simulink model "passThrough"  (R2023a)
settings: Solver=FixedStepDiscrete  StartTime=0.0  StopTime=100  RelTol=1e-3
InitFcn:
  | xlEvaluateHDLBlocks('passThrough')
undefined symbols (not defined in the file): S, vsva2197, xcvc1902
libraries: aieUtilities x2, hdlUtilities x2, aieBasic x1, simulink x1, hdlBasic x1, dspsrcs4 x1, vmcUtilities x1
settings Model: Creator=shirazi  LastModifiedBy=robg
settings SolverCC: AlgebraicLoopSolver=TrustRegion
settings DebuggingCC: UnconnectedInputMsg=warning  UnconnectedOutputMsg=warning  UnconnectedLineMsg=warning
settings ModelReferenceCC: EnableRefExpFcnMdlSchedulingChecks=on
settings SFSimCC: CustomCodeUndefinedFunction=UseInterfaceOnly
settings RTWCC: DLArmComputeVersion=19.05

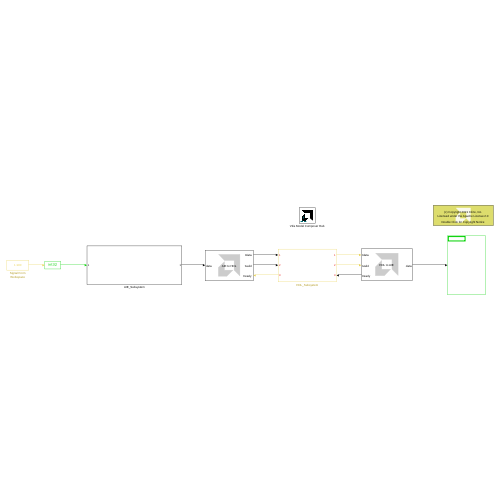
[thumbnail: Simulink's stored preview of the top-level diagram]
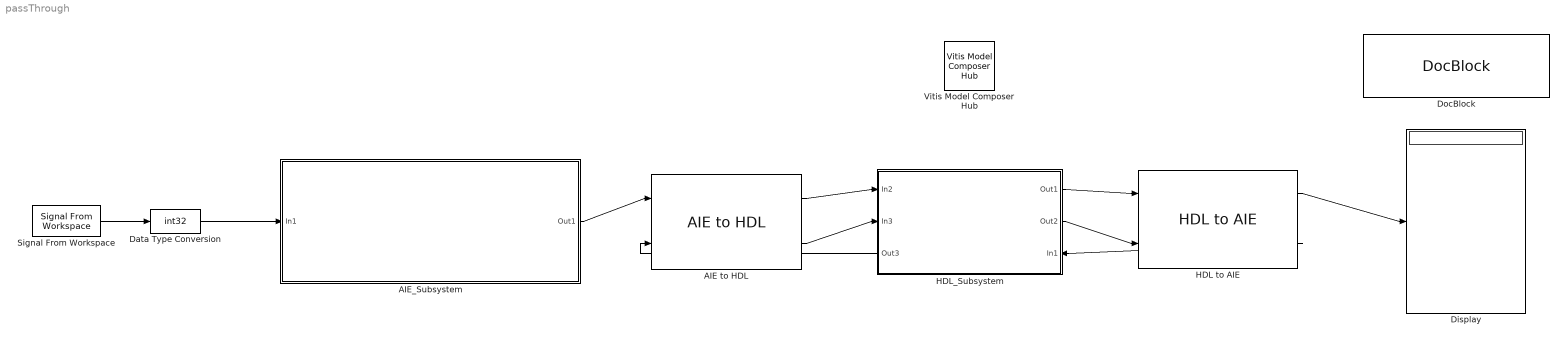
== system passThrough ==
  AIE to HDL : aieUtilities/AIE to HDL  OutDataType=int32  OutSampleTime=Inherit: Same as tready
  AIE_Subsystem : Subsystem
  Data Type Conversion : DataTypeConversion  OutDataTypeStr=int32  SaturateOnIntegerOverflow=off  RndMeth=Floor
  Display : Display
  DocBlock : simulink/Model-Wide Utilities/DocBlock  DocumentType=Text  mask(DocBlock){}
      content=|
      | ///////////////////////////////////////////////////////////////////////////
      | // Copyright 2021 Xilinx
      | //
      | // Licensed under the Apache License, Version 2.0 (the "License");
      | // you may not use this file except in compliance with the License.
      | // You may obtain a copy of the License at
      | //
      | // http://www.apache.org/licenses/LICENSE-2.0
      | //
      | // Unless required by applicable law or agreed to in writing, software
      | // distributed under the License is distributed on an "AS IS" BASIS,
      | // WITHOUT WARRANTIES OR CONDITIONS OF ANY KIND, either express or implied.
      | // See the License for the specific language governing permissions and
      | // limitations under the License.
      | ///////////////////////////////////////////////////////////////////////////
      mask Display:
      | xmcDrawBlockIcon();
      | disp(['{\fontsize{10pt}(c) Copyright 2021' ' Xilinx, Inc.}\newline \newline '],'texmode','on');
      | disp('{\fontsize{10pt}Licensed under the Apache License 2.0}','texmode','on');
      | disp('\newline \newline \newline{\fontsize{10pt}Double Click for Copyright Notice}','texmode','on');
  HDL to AIE : aieUtilities/HDL to AIE  InDataType=uint32  OutDataType=int32  OutSampleTime=1  SamplesPerFrame=8  RateReduceFactor=1  ManuallySpecifyOutSampleTime=on
  HDL_Subsystem : Subsystem
      settings: PortSchema="{\"entries\":[{\"content\":{\"sides\":[{\"content\":{\"connectorIds\":[\"In1\",\"In2\",\"Out3\"]},\"type\":\"ConnectorPlacement.EquallySpacedRectSide\",\"uuid\":\"989cb16a-31ef-4a7b-a4d3-adb9fa6297fb\"},{\"content\":{\"connectorIds\":[\"Out1\",\"Out2\",\"In3\"],\"side\":\"RIGHT\"},\"type\":\"ConnectorPlacement.EquallySpacedRectSide\",\"uuid\":\"9f541dfa-b9f2-4468-aad7-758d6944575e\"},{\"content\":{\"connectorIds\":[],\"side\":\"TOP\"},\"type\":\"ConnectorPlacement.EquallySpacedRectSide\",\"uuid\":\"c3c29352-583e-46d2-970b-15c15d07c124\"}]},\"type\":\"ConnectorPlacement.EquallySpacedConnector\",\"uuid\":\"c80158a0-6c2e-4236-83b1-850c61320738\"}],\"packageUris\":[\"http://schema.mathworks.com/mf0/Connector/19700101\"],\"version\":\"1.0\"}"
  Signal From Workspace : dspsrcs4/Signal From Workspace  X=1:100  Ts=1  nsamps=8  OutputAfterFinalValue=Cyclic repetition  ignoreOrWarnInputAndFrameLengths=off  OutputFrames=off
  Vitis Model Composer Hub : vmcUtilities/Vitis Model Composer Hub  Tag=genX  CodeGeneration=off  SubsystemName=AIE_Subsystem  StartColumn=1  NumberOfColumns=1  TargetDirectory=./code  exportDesign=off  analyzeDesign=off  validateDesignOnHw=off  ExportType=AI Engines  IpVendor=xilinx.com  IpLibrary=hls  IpVersion=1.0  IpHWLanguage=Verilog  AieCompilerOptions={}  AieSimulatorOptions={}  CreateTestbench=off  TestbenchStackSize=10  RunRtlSim=off  RunCSim=off  RunAieSim=off  AieSimTimeout=50000  RunAieSimProfiling=off  LaunchVitisAnalyzer=off  PlotOutput=off  RunX86Sim=off  X86SimTimeout=10  GenHwImage=off  GenLibadfXo=off  GenHwValidationCode=off  PlatformType=Not Specified  HwSystemType=Baremetal  HwValidationTarget=hw  ProjDevice=xcvc1902-vsva2197-1LP-e-S  ProjDevicePart=xcvc1902-vsva2197-1LP-e-S  AIEType=AIE  SamplePeriod=-1  ClockFrequency=200  DataPathParallelism=1  xilinxfamily=versalaicore  part=xcvc1902  speed=-1LP-e-S  package=vsva2197  directory=./netlist  testbench=off  incr_netlist=off  synthesis_tool=Vivado  clock_wrapper=Clock Enables  dbl_ovrd=According to Block Masks  dcm_input_clock_period=10  sysclk_period=10  simulink_period=1  eval_field=0  LogFileName=''  NThreads=4
  wires:
  Signal From Workspace/1 -> Data Type Conversion/1
  HDL to AIE/1 -> Display/1
  HDL_Subsystem/1(Out1) -> HDL to AIE/1
  AIE to HDL/1 -> HDL_Subsystem/1(In2)
  HDL_Subsystem/2(Out2) -> HDL to AIE/2
  AIE to HDL/2 -> HDL_Subsystem/2(In3)
  HDL to AIE/2 -> HDL_Subsystem/3(In1)
  HDL_Subsystem/3(Out3) -> AIE to HDL/2
  Data Type Conversion/1 -> AIE_Subsystem/1(In1)
  AIE_Subsystem/1(Out1) -> AIE to HDL/1

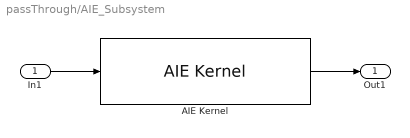
== system passThrough/AIE_Subsystem ==
  In1 : Inport
  AIE Kernel : aieBasic/AIE Kernel  KernelAllAttrs=s[12;12;9;9;19;14;21;23;24;21;12;24;26;26;26;27;28;9;21;23;23;23;24;25;14;19;19;29]@FunctionNameDeclFileNamePortNamesPortTypesPortSerializedTypesPortDirectionsPortWindowSizeEnablesPortWindowMarginEnablesPortSynchronicityEnablesPortSignalSizeEnablesFunctionDeclFunctionTemplateSpecKindFunctionTemplateParamNamesFunctionTemplateParamKindsFunctionTemplateParamTypesFunctionTemplateParamValuesFunctionTemplateParamEnablesClassDeclClassTemplateSpecKindClassTemplateParamNamesClassTemplateParamKindsClassTemplateParamTypesClassTemplateParamValuesClassTemplateParamEnablesClassCtorDeclsClassCtorParamNamesClassCtorParamTypesClassCtorParamSerializedTypes[1 1]@C[28 1]@t8@mysquaret16@../../mysquare.hC[2 1]@t3@in1t4@out1C[2 1]@t20@input_window_int32 *t21@output_window_int32 *C[2 1]@t30@{P{Tinput_window{1{t{Bi32}}}}}t31@{P{Toutput_window{1{t{Bi32}}}}}C[2 1]@t5@inputt6@outputC[2 1]@l1@l1@C[2 1]@l1@l0@C[2 1]@l1@l1@C[2 1]@l0@l0@t67@void mysquare(input_window_int32 * in1, output_window_int32 * out1)t4@nonee[0 1]@e[0 1]@e[0 1]@e[0 1]@e[0 1]@nne[0 1]@e[0 1]@e[0 1]@e[0 1]@e[0 1]@e[0 1]@e[0 1]@e[0 1]@e[0 1]@  PortNames={'in1'; 'out1'}  PortSerializedTypes={'{P{Tinput_window{1{t{Bi32}}}}}'; '{P{Toutput_window{1{t{Bi32}}}}}'}  PortWindowSizes={8.000000000000000000e+00, 8.000000000000000000e+00}  PortWindowMargins={0.000000000000000000e+00, 0.000000000000000000e+00}  PortSynchronicities={'sync', 'sync'}  PortSignalSizes={0.000000000000000000e+00; 0.000000000000000000e+00}  FunctionTemplateSpecKind=none  FunctionTemplateParamNames={}  FunctionTemplateParamKinds={}  FunctionTemplateParamTypes={}  FunctionTemplateParamValues={}  FunctionIndex=1  FunctionTabVisible=on  FunctionTemplateParamsVisible=off  FunctionDeclTypeOptions=C[1 1]@t70@void mysquare(input_window_int32 * _arg0, output_window_int32 * _arg1)  FunctionDecl=void mysquare(input_window_int32 * _arg0, output_window_int32 * _arg1)  FunctionTemplateParams={}  FunctionTemplateParamsEnables={}  PortAttrs={ 'Input', '_arg0', 'input_window_int32 *', '8', '0', 'sync', ''; 'Output', '_arg1', 'output_window_int32 *', '8', '', 'sync', '' }  PortAttrsEnables={'off', 'off', 'off', 'on', 'on', 'on', 'off';'off', 'off', 'off', 'on', 'off', 'on', 'off'}  SampleTime=-1  KernelHeaderFile=mysquare.h  KernelFunction=mysquare  KernelSourceFile=mysquare.cc  KernelSearchPaths={}  PreProcOptions={}  blockJsonConstraints=[]
  Out1 : Outport
  wires:
  In1/1 -> AIE Kernel/1
  AIE Kernel/1 -> Out1/1

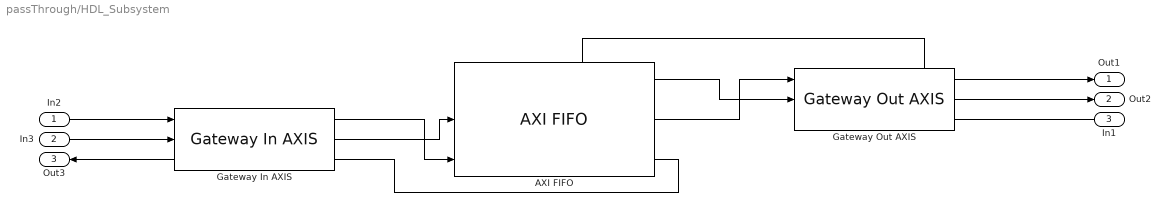
== system passThrough/HDL_Subsystem ==
  In2 : Inport
  In3 : Inport  Port=2
  In1 : Inport  Port=3
  AXI FIFO : hdlBasic/AXI FIFO  input_depth_axis=1K  actual_fifo_depth_label=1026  enable_tdata=on  enable_tdest=off  enable_tstrb=off  enable_tready=on  enable_tid=off  enable_tuser=off  enable_tkeep=off  enable_tlast=off  has_aresetn=off  enable_data_counts_axis=off  fifo_implementation_type_axis=Common Clock Block RAM  trim_axipin_name=off  programmable_full_type_axis=Full  full_threshold_assert_value_axis=0  programmable_empty_type_axis=Empty  empty_threshold_assert_value_axis=1022  underflow_flag_axi=0  underflow_sense_axi=Active High  overflow_flag_axi=0  overflow_sense_axi=Active High  simulation_type=fast_sim  XmcBlockStatus=1  maskContainerNames=tabcontainer1  block_type=axi_fifo  block_config=sysgen:AXI_FIFO_config
  Gateway In AXIS : hdlUtilities/Gateway In AXIS  gui_display_data_type=Fixed-point  arith_type=Signed (2's comp)  n_bits=32  bin_pt=0  preci_type=Custom  exp_width=16  frac_width=24  quantization=Truncate  overflow=Flag as error  OutSampleTime=1  block_type=gatewayinaxi  XmcBlockStatus=1
  Gateway Out AXIS : hdlUtilities/Gateway Out AXIS  mask_sample_period=1  block_type=gatewayoutaxi
  Out1 : Outport
  Out2 : Outport  Port=2
  Out3 : Outport  Port=3
  wires:
  AXI FIFO/2 -> Gateway Out AXIS/1
  AXI FIFO/1 -> Gateway Out AXIS/2
  In1/1 -> Gateway Out AXIS/3
  AXI FIFO/3 -> Gateway In AXIS/3
  In3/1 -> Gateway In AXIS/2
  In2/1 -> Gateway In AXIS/1
  Gateway Out AXIS/3 -> AXI FIFO/1
  Gateway In AXIS/3 -> Out3/1
  Gateway Out AXIS/2 -> Out2/1
  Gateway Out AXIS/1 -> Out1/1
  Gateway In AXIS/1 -> AXI FIFO/3
  Gateway In AXIS/2 -> AXI FIFO/2
